simulink model "fengji"  (R2022b)
settings: Solver=VariableStepAuto  StartTime=0.0  StopTime=1.2  RelTol=1e-3
InitFcn:
  | Udc=311;
  | R=0.958;
  | Ld=5.25e-3;
  | Lq=12e-3;
  | flux=0.1827;
  | J=0.003;
  | B=0.008;
  | Pn=4;
  | Kpd=1100*0.958;
  | Kid=1100*R;
  | Kpq=1100*Lq;
  | Kiq=1100*R;
  | uppermin=-311*0.9*sqrt(1/3);
  | uppermax=311*0.9*sqrt(1/3);
  | uppermin2=-311*0.9*sqrt(1/3);
  | uppermax2=311*0.9*sqrt(1/3);
  | Kpw=0.14;
  | Kiw=0.14*50;
  | Ba=0.013;
undefined symbols (not defined in the file): DiscIntNeverNeededParam
libraries: simulink x11, slpidlib x6, spsabctodq0Lib x3, spsUniversalBridgeLib x3, spsPermanentMagnetSynchronousMachineLib x2, spsSVPWMGenerator2LevelLib x2, spsdq0toAlphaBetaZeroLib x2, spsPower3phInstantaneousLib x1, spsPower3phPhasorLib x1, spsSeriesRLCBranchLib x1, spsDCVoltageSourceLib x1, spsThreePhaseSeriesRLCBranchLib x1
(part 2 of 2)

== system fengji/Subsystem7/svpwm'/Subsystem4 ==
  T1' : Inport
  T2' : Inport  Port=2
  Tpwm : Inport  Port=3
  Add : Sum  Inputs=+--
  Add1 : Sum
  Add2 : Sum
  Gain : Gain  Gain=1/4
  Gain1 : Gain  Gain=1/2
  Gain2 : Gain  Gain=1/2
  Ta : Outport
  Tb : Outport  Port=2
  Tc : Outport  Port=3
  wires:
  Gain1/1 -> Add1/2
  T1'/1 -> Gain1/1, Add/2
  Gain2/1 -> Add2/2
  Add1/1 -> Tb/1, Add2/1
  Gain/1 -> Ta/1, Add1/1
  Add/1 -> Gain/1
  Tpwm/1 -> Add/1
  T2'/1 -> Gain2/1, Add/3
  Add2/1 -> Tc/1

== system fengji/Subsystem7/svpwm'/Subsystem5 ==
  N : Inport
  Ta : Inport  Port=2
  Tb : Inport  Port=3
  Tc : Inport  Port=4
  Multiport Switch1 : MultiPortSwitch  Inputs=6  SaturateOnIntegerOverflow=off  InputSameDT=off
  Multiport Switch2 : MultiPortSwitch  Inputs=6  SaturateOnIntegerOverflow=off  InputSameDT=off
  Multiport Switch3 : MultiPortSwitch  Inputs=6  SaturateOnIntegerOverflow=off  InputSameDT=off
  Tcmp1 : Outport
  Tcmp2 : Outport  Port=2
  Tcmp3 : Outport  Port=3
  wires:
  Multiport Switch1/1 -> Tcmp1/1
  N/1 -> Multiport Switch1/1, Multiport Switch3/1, Multiport Switch2/1
  Tb/1 -> Multiport Switch3/6, Multiport Switch2/5, Multiport Switch2/4, Multiport Switch1/7, Multiport Switch1/2, Multiport Switch3/3
  Multiport Switch3/1 -> Tcmp3/1
  Tc/1 -> Multiport Switch3/4, Multiport Switch3/2, Multiport Switch2/7, Multiport Switch2/3, Multiport Switch1/6, Multiport Switch1/5
  Ta/1 -> Multiport Switch3/5, Multiport Switch3/7, Multiport Switch2/6, Multiport Switch2/2, Multiport Switch1/4, Multiport Switch1/3
  Multiport Switch2/1 -> Tcmp2/1

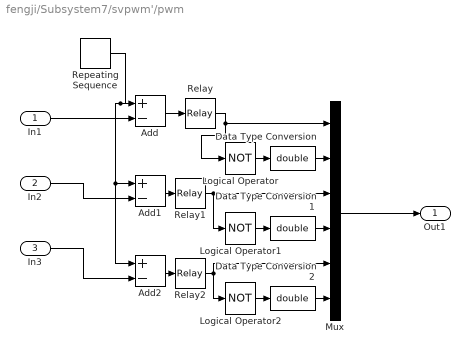
== system fengji/Subsystem7/svpwm'/pwm ==
  In1 : Inport
  In2 : Inport  Port=2
  In3 : Inport  Port=3
  Add : Sum  Inputs=+-
  Add1 : Sum  Inputs=+-
  Add2 : Sum  Inputs=+-
  Data Type Conversion : DataTypeConversion  OutDataTypeStr=double  SaturateOnIntegerOverflow=off  RndMeth=Floor
  Data Type Conversion1 : DataTypeConversion  OutDataTypeStr=double  SaturateOnIntegerOverflow=off  RndMeth=Floor
  Data Type Conversion2 : DataTypeConversion  OutDataTypeStr=double  SaturateOnIntegerOverflow=off  RndMeth=Floor
  Logical Operator : Logic  Operator=NOT  AllPortsSameDT=off  OutDataTypeStr=boolean
  Logical Operator1 : Logic  Operator=NOT  AllPortsSameDT=off  OutDataTypeStr=boolean
  Logical Operator2 : Logic  Operator=NOT  AllPortsSameDT=off  OutDataTypeStr=boolean
  Mux : Mux  Inputs=6
  Relay : Relay
  Relay1 : Relay
  Relay2 : Relay
  Repeating Sequence : simulink/Sources/Repeating Sequence  rep_seq_t=[0 0.5 1]*10e-5  rep_seq_y=[0 0.5 0]*10e-5
  Out1 : Outport
  wires:
  Add2/1 -> Relay2/1
  Relay/1 -> Logical Operator/1, Mux/1
  Relay2/1 -> Logical Operator2/1, Mux/5
  Relay1/1 -> Logical Operator1/1, Mux/3
  Logical Operator2/1 -> Data Type Conversion2/1
  Repeating Sequence/1 -> Add2/1, Add1/1, Add/1
  Data Type Conversion1/1 -> Mux/4
  Add1/1 -> Relay1/1
  Add/1 -> Relay/1
  Logical Operator1/1 -> Data Type Conversion1/1
  Data Type Conversion/1 -> Mux/2
  Data Type Conversion2/1 -> Mux/6
  In1/1 -> Add/2
  Logical Operator/1 -> Data Type Conversion/1
  In2/1 -> Add1/2
  In3/1 -> Add2/2
  Mux/1 -> Out1/1

== matlab function fengji/fengliji/MATLAB Function ==
  data: u input; y output
function y = fcn(u)
u=0.5*pi*u(2)^2*u(1)*u(3)^3*u(4)
y = u;

== matlab function fengji/fengliji/MATLAB Function2 ==
  data: u input; y output
function y = fcn(u)
u=1/(u(1)+0.08*u(2))-(0.035/(u(2)^3+1))
y = u;

== matlab function fengji/Subsystem7/anti_park/MATLAB Function ==
  data: u input; y output
function y = fcn(u)
u=cos(u(1))*u(2)-sin(u(1))*u(3);
y = u;

== matlab function fengji/Subsystem7/anti_park/MATLAB Function1 ==
  data: u input; y output
function y = fcn(u)
u=sin(u(1))*u(2)+cos(u(1))*u(3);
y = u;

== matlab function fengji/Subsystem7/clark/MATLAB Function ==
  data: u input; y output
function y = fcn(u)
u=2/3*(u(1)-0.5*(u(2)+u(3)));
y = u;

== matlab function fengji/Subsystem7/clark/MATLAB Function1 ==
  data: u input; y output
function y = fcn(u)
u=2/3*(sqrt(3)/2*(u(2)-u(3)));
y = u;

== matlab function fengji/Subsystem7/park/MATLAB Function ==
  data: u input; y output
function y = fcn(u)
u=u(1)*cos(u(3))+u(2)*sin(u(3));
y = u;

== matlab function fengji/Subsystem7/park/MATLAB Function1 ==
  data: u input; y output
function y = fcn(u)
u=-u(1)*sin(u(3))+u(2)*cos(u(3));
y = u;

== matlab function fengji/fengliji/MATLAB Function1 ==
  data: u input; y output
function y = fcn(u)
u=0.5176*(116*u(2)-0.4*u(3)-5)*exp(-21*u(2))+0.0068*u(1)
y = u;
